simulink model "Lab6_2"  (R2016a)
settings: Solver=VariableStepAuto  StartTime=0.0  StopTime=10.0  RelTol=1e-3
settings Model: Creator=Student  LastModifiedBy=Student

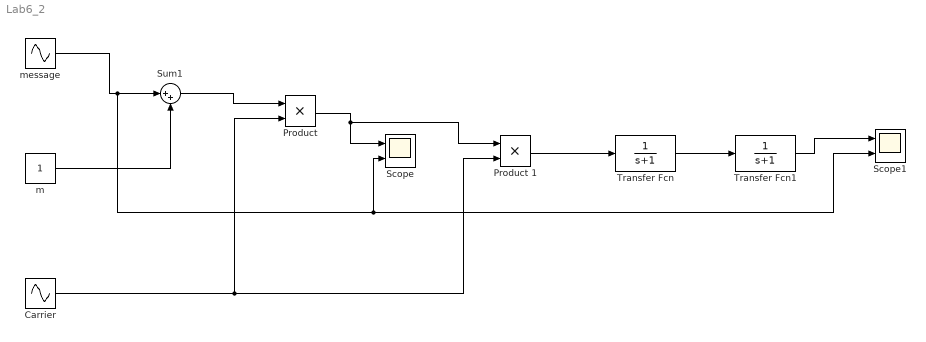
== system Lab6_2 ==
  Carrier : Sin  Amplitude=5  Frequency=2*pi*25  SampleTime=1/5000
  "Product " : Product
  Product 1 : Product
  Scope : Scope  NumInputPorts=2
  Scope1 : Scope  NumInputPorts=2
  Sum1 : Sum  Inputs=|++
  Transfer Fcn : TransferFcn  Denominator=[1 1]
  Transfer Fcn1 : TransferFcn  Denominator=[1 1]
  m : Constant
  message : Sin  Frequency=2*pi  SampleTime=1/5000
  wires:
  Carrier/1 -> Product 1/2, "Product "/2
  m/1 -> Sum1/2
  message/1 -> Scope/2, Scope1/2, Sum1/1
  Sum1/1 -> "Product "/1
  "Product "/1 -> Product 1/1, Scope/1
  Product 1/1 -> Transfer Fcn/1
  Transfer Fcn/1 -> Transfer Fcn1/1
  Transfer Fcn1/1 -> Scope1/1
